simulink model "DTFC_SVM"  (R2019b)
settings: Solver=VariableStepAuto  StartTime=0.0  StopTime=15  RelTol=1e-3
undefined symbols (not defined in the file or in its folder): find_system, psisx, Rs, Ts, Ts_SVPWM, Vdc
libraries: powerlib x15, powerlib_meascontrol x3, simulink_extras x3, simulink x2
settings Model: Creator=ADHI  LastModifiedBy=ADHI
settings DataIOCC: ReturnWorkspaceOutputs=off
settings DebuggingCC: ArithmeticOperatorsInVariantConditions=warning
settings SFSimCC: SimUseLocalCustomCode=off  CustomCodeUndefinedFunction=UseInterfaceOnly
settings RTWCC: RTWUseLocalCustomCode=off

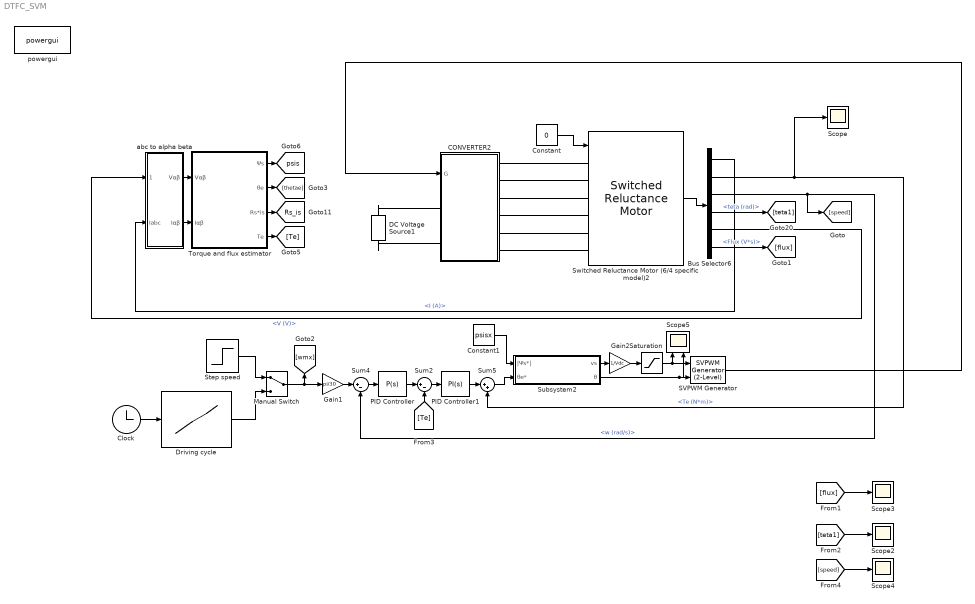
== system DTFC_SVM ==
  Bus Selector6 : BusSelector  OutputSignals=I (A),Te (N*m),w (rad/s),teta (rad),V (V),Flux (V*s)
  CONVERTER2 : Subsystem  LoadFcn=find_system(gcs,'FollowLinks', 'on', 'LookUnderMasks', 'all');
  Clock : Clock
  Constant : Constant  Value=0
  Constant1 : Constant  Value=psisx
  DC Voltage Source1 : powerlib/Electrical Sources/DC Voltage Source  Amplitude=250  Measurements=None
      settings: SourceProductName=Simscape Electrical
  Driving cycle : Lookup_n-D  NumberOfTableDimensions=1  BreakpointsForDimension1=[0 1 2 5 5.001 8 8.001 10 11 12]/2  Table=[0 0 480 480 1430 1430 0 0 480 480]  RndMeth=Simplest  InputSameDT=on
  Gain1 : Gain  Gain=pi/30
  Gain2 : Gain  Gain=1/Vdc
  Manual Switch : ManualSwitch
  PID Controller : simulink/Continuous/PID Controller  Controller=P  Form=Parallel  TimeDomain=Continuous-time  SampleTime=-1  IntegratorMethod=Forward Euler  FilterMethod=Forward Euler  ControllerParametersSource=internal  P=20  I=20  D=0  UseFilter=on  N=100  TunerSelectOption=Transfer Function Based (PID Tuner App)  InitialConditionSource=internal  InitialConditionForIntegrator=0  InitialConditionForFilter=0  DifferentiatorICPrevScaledInput=0  ExternalReset=none  TrackingMode=off  Kt=1  LimitOutput=on  UpperSaturationLimit=30  LowerSaturationLimit=-30  LinearizeAsGain=on  AntiWindupMode=clamping  Kb=1  POutMin=[]  POutMax=[]  IOutMin=[]  IOutMax=[]  DOutMin=[]  DOutMax=[]  NOutMin=[]  NOutMax=[]  SumOutMin=[]  SumOutMax=[]  SaturationOutMin=[]  SaturationOutMax=[]  PParamMin=[]  PParamMax=[]  IParamMin=[]  IParamMax=[]  DParamMin=[]  DParamMax=[]  NParamMin=[]  NParamMax=[]  KbParamMin=[]  KbParamMax=[]  KtParamMin=[]  KtParamMax=[]  KbOutMin=[]  KbOutMax=[]  KtOutMin=[]  KtOutMax=[]  IntegratorOutMin=[]  IntegratorOutMax=[]  FilterOutMin=[]  FilterOutMax=[]  SumI1OutMin=[]  SumI1OutMax=[]  SumI2OutMin=[]  SumI2OutMax=[]  SumI3OutMin=[]  SumI3OutMax=[]  SumI4OutMin=[]  SumI4OutMax=[]  SumDOutMin=[]  SumDOutMax=[]  DifferentiatorOutMin=[]  DifferentiatorOutMax=[]  FilterDiffOutCoefMin=[]  FilterDiffOutCoefMax=[]  ReciprocalOutMin=[]  ReciprocalOutMax=[]  SumDenOutMin=[]  SumDenOutMax=[]  SumNumOutMin=[]  SumNumOutMax=[]  DivideOutMin=[]  DivideOutMax=[]  IntegratorContinuousStateAttributes=''  IntegratorStateMustResolveToSignalObject=off  IntegratorRTWStateStorageClass=Auto  FilterContinuousStateAttributes=''  FilterStateMustResolveToSignalObject=off  FilterRTWStateStorageClass=Auto  ParallelPVariant=InternalParameters  IdealPVariant=Disabled  IVariant=Disabled  DVariant=Disabled  IntegratorVariant=Disabled  SatVariant=Enabled  AWVariant=Disabled  PCopyVariant=Disabled  TRVariant=Disabled  FdbkBlocksVariant=Forward  IdealPFdbkVariant=Disabled  SatFdbkVariant=Disabled  DerivativeFilterVariant=Disabled  NVariant=Disabled  NCopyVariant=Disabled_SignalSpec  FilterICVariant=Disabled  IntegratorICVariant=Disabled  ExternalResetVariant=Disabled  TRSumVariant=Passthrough  SumFdbkVariant=Disabled  SumVariant=Passthrough_P
  PID Controller1 : simulink/Continuous/PID Controller  Controller=PI  Form=Parallel  TimeDomain=Continuous-time  SampleTime=-1  IntegratorMethod=Forward Euler  FilterMethod=Forward Euler  ControllerParametersSource=internal  P=0.005  I=1  D=0.00005  UseFilter=on  N=100  TunerSelectOption=Transfer Function Based (PID Tuner App)  InitialConditionSource=internal  InitialConditionForIntegrator=0  InitialConditionForFilter=0  DifferentiatorICPrevScaledInput=0  ExternalReset=none  TrackingMode=off  Kt=1  LimitOutput=on  UpperSaturationLimit=pi/2  LowerSaturationLimit=-pi/2  LinearizeAsGain=on  AntiWindupMode=clamping  Kb=1  POutMin=[]  POutMax=[]  IOutMin=[]  IOutMax=[]  DOutMin=[]  DOutMax=[]  NOutMin=[]  NOutMax=[]  SumOutMin=[]  SumOutMax=[]  SaturationOutMin=[]  SaturationOutMax=[]  PParamMin=[]  PParamMax=[]  IParamMin=[]  IParamMax=[]  DParamMin=[]  DParamMax=[]  NParamMin=[]  NParamMax=[]  KbParamMin=[]  KbParamMax=[]  KtParamMin=[]  KtParamMax=[]  KbOutMin=[]  KbOutMax=[]  KtOutMin=[]  KtOutMax=[]  IntegratorOutMin=[]  IntegratorOutMax=[]  FilterOutMin=[]  FilterOutMax=[]  SumI1OutMin=[]  SumI1OutMax=[]  SumI2OutMin=[]  SumI2OutMax=[]  SumI3OutMin=[]  SumI3OutMax=[]  SumI4OutMin=[]  SumI4OutMax=[]  SumDOutMin=[]  SumDOutMax=[]  DifferentiatorOutMin=[]  DifferentiatorOutMax=[]  FilterDiffOutCoefMin=[]  FilterDiffOutCoefMax=[]  ReciprocalOutMin=[]  ReciprocalOutMax=[]  SumDenOutMin=[]  SumDenOutMax=[]  SumNumOutMin=[]  SumNumOutMax=[]  DivideOutMin=[]  DivideOutMax=[]  IntegratorContinuousStateAttributes=''  IntegratorStateMustResolveToSignalObject=off  IntegratorRTWStateStorageClass=Auto  FilterContinuousStateAttributes=''  FilterStateMustResolveToSignalObject=off  FilterRTWStateStorageClass=Auto  ParallelPVariant=InternalParameters  IdealPVariant=Disabled  IVariant=InternalParameters  DVariant=Disabled  IntegratorVariant=Continuous  SatVariant=Enabled  AWVariant=ContClampingParallel  PCopyVariant=Disabled  TRVariant=Disabled  FdbkBlocksVariant=Forward  IdealPFdbkVariant=Disabled  SatFdbkVariant=Disabled  DerivativeFilterVariant=Disabled  NVariant=Disabled  NCopyVariant=Disabled_SignalSpec  FilterICVariant=Disabled  IntegratorICVariant=InternalICs  ExternalResetVariant=Disabled  TRSumVariant=Passthrough  SumFdbkVariant=Disabled  SumVariant=Sum_PI
  SVPWM Generator : powerlib_meascontrol/Pulse & Signal Generators/SVPWM Generator (2-Level)  InputType=Magnitude-Angle (rad)  SwitchingPattern=Pattern #1  Fc=1/Ts_SVPWM  ParUref=[0.8 -30 50]  Ts=Ts
      settings: SourceProductName=Simscape Electrical  SourceProductBaseCode=PS
  Saturation : Saturate  UpperLimit=1  LowerLimit=0
  Scope{,2..4} (4 alike) : Scope
  Scope5 : Scope  NumInputPorts=2
  Step speed : Step  Time=0.15  After=1200  SampleTime=0
  Subsystem2 : Subsystem
  Sum2 : Sum  Inputs=|+-
  Sum4 : Sum  Inputs=|+-  SaturateOnIntegerOverflow=on  InputSameDT=on  OutDataTypeStr=Inherit: Same as first input
  Sum5 : Sum  Inputs=|++
  Switched Reluctance Motor (6/4 specific model)2 : powerlib/Machines/Switched Reluctance Motor  MachineType=6/4  StatorResistance=0.05  Inertia=0.05  Friction=0.02  InitialSpeed=[0,0]  TsPowergui=0  TsBlock=Ts  MachineModel=Specific model  Lq=0.67e-3  Ld=23.6e-3  Lsat=0.15e-3  MaximumCurrent=450  MaximumFluxLinkage=0.486  Source=Dialog  MagnetisationCharacteristic=FTBL  RotorAngleVector=RotorAngles  StatorCurrentVector=StatorCurrents  PlotCurves=off
      settings: SourceProductName=Simscape Electrical  SourceProductBaseCode=PS
  Torque and flux estimator : Subsystem
  abc to alpha beta : Subsystem
  powergui : powerlib/powergui  Priority=1  SimulationMode=Discrete  SampleTime=Ts  frequency=60  Iterations=50  frequencyindice=0  Pbase=100e6  ErrMax=1e-4  UnitsV=kV  UnitsW=MW  buscounter=0  FunctionMessages=off  echomessages=off  EnableUseOfTLC=off  CurrentSourceSwitches=off  DisableSnubberDevices=off  DisableRonSwitches=off  DisableVfSwitches=off  DisplayEquations=off  AutomaticDiscreteSolvers=off  SolverType=Tustin/Backward Euler (TBE)  Interpol=off  ExternalGateDelay=off  methode=off  Ts=100  x0status=blocks  SPID=off  SwTol=0  HookPort=off  NonlinearTolerance=1e-4  nMaxIteration=100  ContinueOnMaxIteration=off  RestoreLinks=warning  ResistiveCurrentMeasurement=off  Frange=[0:2:500]  Ylog=off  Xlog=on  ShowGrid=off  save=off  variable=ZData  structure=0  ZoomFFT=off  StartTime=0.0  cycles=1  DisplayStyle=1  fundamental=60  FreqAxis=off  MaxFrequency=1000  frequencyindicesteady=1  RmsSteady=1  display=off
      settings: SourceProductName=Simscape Electrical
  tag scope: Rs_is=global, psis=global
  wires:
  SVPWM Generator/1 -> CONVERTER2/1(G)
  Switched Reluctance Motor (6/4 specific model)2/1 -> Bus Selector6/1
  Bus Selector6/1 -> abc to alpha beta/2(Iabc)  "<I (A)>"
  Bus Selector6/5 -> abc to alpha beta/1(Vabc)  "<V (V)>"
  Bus Selector6/4 -> [teta1]  "<teta (rad)>"
  Bus Selector6/3 -> [speed], Sum4/2  "<w (rad/s)>"
  Bus Selector6/2 -> Scope/1, Sum5/2  "<Te (N*m)>"
  Gain2/1 -> Saturation/1
  Sum5/1 -> Subsystem2/2(θe*)
  Sum4/1 -> PID Controller/1
  Torque and flux estimator/2(θe) -> [thetae]
  Driving cycle/1 -> Manual Switch/2
  abc to alpha beta/1(Vαβ) -> Torque and flux estimator/1(Vαβ)
  Torque and flux estimator/4(Te) -> [Te]
  Clock/1 -> Driving cycle/1
  Torque and flux estimator/1(Ψs) -> [psis]
  Torque and flux estimator/3(Rs*is) -> [Rs_is]
  Sum2/1 -> PID Controller1/1
  Constant1/1 -> Subsystem2/1(|Ψs*|)
  [Te] -> Sum2/2
  Subsystem2/1(vs) -> Gain2/1
  PID Controller1/1 -> Sum5/1
  Gain1/1 -> Sum4/1
  Manual Switch/1 -> [wmx], Gain1/1
  abc to alpha beta/2(Iαβ) -> Torque and flux estimator/2(Iαβ)
  Step speed/1 -> Manual Switch/1
  Saturation/1 -> SVPWM Generator/1, Scope5/1
  PID Controller/1 -> Sum2/1
  Subsystem2/2(θ) -> Scope5/2, SVPWM Generator/2
  Constant/1 -> Switched Reluctance Motor (6/4 specific model)2/1
  Bus Selector6/6 -> [flux]  "<Flux (V*s)>"
  [flux] -> Scope3/1
  [teta1] -> Scope2/1
  [speed] -> Scope4/1
  connections:
  CONVERTER2/RConn1 -- Switched Reluctance Motor (6/4 specific model)2/LConn1
  CONVERTER2/RConn2 -- Switched Reluctance Motor (6/4 specific model)2/LConn2
  CONVERTER2/RConn3 -- Switched Reluctance Motor (6/4 specific model)2/LConn3
  CONVERTER2/RConn4 -- Switched Reluctance Motor (6/4 specific model)2/LConn4
  CONVERTER2/RConn5 -- Switched Reluctance Motor (6/4 specific model)2/LConn5
  CONVERTER2/RConn6 -- Switched Reluctance Motor (6/4 specific model)2/LConn6
  DC Voltage Source1/RConn1 -- CONVERTER2/LConn1
  DC Voltage Source1/LConn1 -- CONVERTER2/LConn2

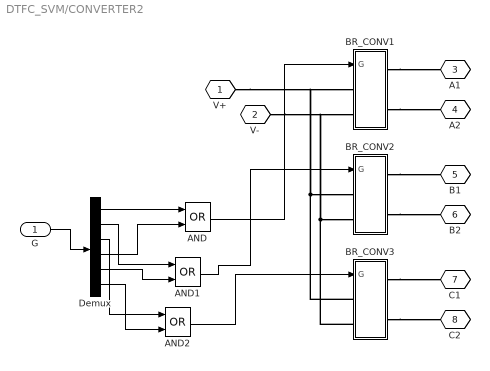
== system DTFC_SVM/CONVERTER2 ==
  G : Inport
  AND : Logic  Operator=OR  AllPortsSameDT=off  OutDataTypeStr=boolean
  AND1 : Logic  Operator=OR  AllPortsSameDT=off  OutDataTypeStr=boolean
  AND2 : Logic  Operator=OR  AllPortsSameDT=off  OutDataTypeStr=boolean
  BR_CONV1 : Subsystem
  BR_CONV2 : Subsystem
  BR_CONV3 : Subsystem
  Demux : Demux  Outputs=6
  V+ : PMIOPort  Tag=PMCPort  Side=Left
  V- : PMIOPort  Tag=PMCPort  Port=2  Side=Left
  A1 : PMIOPort  Tag=PMCPort  Port=3  Side=Right
  A2 : PMIOPort  Tag=PMCPort  Port=4  Side=Right
  B1 : PMIOPort  Tag=PMCPort  Port=5  Side=Right
  B2 : PMIOPort  Tag=PMCPort  Port=6  Side=Right
  C1 : PMIOPort  Tag=PMCPort  Port=7  Side=Right
  C2 : PMIOPort  Tag=PMCPort  Port=8  Side=Right
  wires:
  G/1 -> Demux/1
  AND/1 -> BR_CONV1/1(G)
  AND1/1 -> BR_CONV2/1(G)
  AND2/1 -> BR_CONV3/1(G)
  Demux/1 -> AND/1
  Demux/4 -> AND/2
  Demux/2 -> AND1/1
  Demux/3 -> AND2/1
  Demux/5 -> AND1/2
  Demux/6 -> AND2/2
  connections:
  BR_CONV3/RConn2 -- C2/RConn1
  BR_CONV3/RConn1 -- C1/RConn1
  BR_CONV2/RConn2 -- B2/RConn1
  BR_CONV2/RConn1 -- B1/RConn1
  BR_CONV1/RConn2 -- A2/RConn1
  BR_CONV1/RConn1 -- A1/RConn1
  BR_CONV3/LConn2 -- BR_CONV1/LConn2 -- V-/RConn1 -- BR_CONV2/LConn2
  BR_CONV3/LConn1 -- BR_CONV1/LConn1 -- V+/RConn1 -- BR_CONV2/LConn1

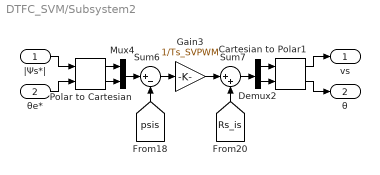
== system DTFC_SVM/Subsystem2 ==
  |Ψs*| : Inport
  θe* : Inport  Port=2
  Cartesian to Polar1 : simulink_extras/Transformations/Cartesian to Polar
      settings: SourceProductName=Simulink
  Demux2 : Demux  Outputs=2
  Gain3 : Gain  Gain=1/Ts_SVPWM
  Mux4 : Mux  Inputs=2
  Polar to Cartesian : simulink_extras/Transformations/Polar to Cartesian
      settings: SourceProductName=Simulink  SourceProductBaseCode=SL
  Sum6 : Sum  Inputs=|+-
  Sum7 : Sum  Inputs=|++
  vs : Outport  VectorParamsAs1DForOutWhenUnconnected=off
  θ : Outport  Port=2  VectorParamsAs1DForOutWhenUnconnected=off
  wires:
  Mux4/1 -> Sum6/1
  |Ψs*|/1 -> Polar to Cartesian/1
  Gain3/1 -> Sum7/1
  Polar to Cartesian/2 -> Mux4/2
  Demux2/1 -> Cartesian to Polar1/1
  Sum6/1 -> Gain3/1
  Demux2/2 -> Cartesian to Polar1/2
  [psis] -> Sum6/2
  Polar to Cartesian/1 -> Mux4/1
  Sum7/1 -> Demux2/1
  [Rs_is] -> Sum7/2
  θe*/1 -> Polar to Cartesian/2
  Cartesian to Polar1/1 -> vs/1
  Cartesian to Polar1/2 -> θ/1

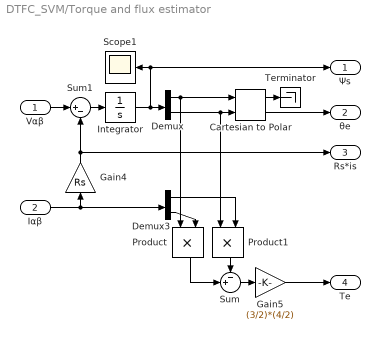
== system DTFC_SVM/Torque and flux estimator ==
  Vαβ : Inport
  Iαβ : Inport  Port=2
  Cartesian to Polar : simulink_extras/Transformations/Cartesian to Polar
      settings: SourceProductName=Simulink
  Demux : Demux  Outputs=2
  Demux3 : Demux  Outputs=2
  Gain4 : Gain  Gain=Rs
  Gain5 : Gain  Gain=(3/2)*(4/2)
  Integrator : Integrator
  Product : Product
  Product1 : Product
  Scope1 : Scope
  Sum : Sum  Inputs=-+|
  Sum1 : Sum  Inputs=|+-
  Terminator : Terminator
  Ψs : Outport  VectorParamsAs1DForOutWhenUnconnected=off
  θe : Outport  Port=2  VectorParamsAs1DForOutWhenUnconnected=off
  Rs*is : Outport  Port=3  VectorParamsAs1DForOutWhenUnconnected=off
  Te : Outport  Port=4  VectorParamsAs1DForOutWhenUnconnected=off
  wires:
  Vαβ/1 -> Sum1/1
  Integrator/1 -> Demux/1, Ψs/1, Scope1/1
  Sum1/1 -> Integrator/1
  Gain4/1 -> Rs*is/1, Sum1/2
  Demux3/1 -> Product1/2
  Demux3/2 -> Product/2
  Demux/2 -> Product1/1, Cartesian to Polar/2
  Product/1 -> Sum/2
  Cartesian to Polar/1 -> Terminator/1
  Demux/1 -> Cartesian to Polar/1, Product/1
  Sum/1 -> Gain5/1
  Product1/1 -> Sum/1
  Iαβ/1 -> Demux3/1, Gain4/1
  Gain5/1 -> Te/1
  Cartesian to Polar/2 -> θe/1

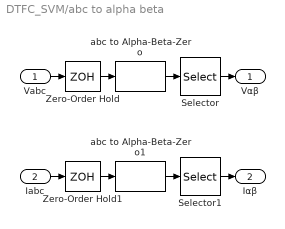
== system DTFC_SVM/abc to alpha beta ==
  Vabc : Inport
  Iabc : Inport  Port=2
  Selector : Selector  InputPortWidth=3  IndexOptions=Index vector (dialog)  Indices=[1 2]  OutputSizes=1
  Selector1 : Selector  InputPortWidth=3  IndexOptions=Index vector (dialog)  Indices=[1 2]  OutputSizes=1
  Zero-Order Hold : ZeroOrderHold  SampleTime=Ts
  Zero-Order Hold1 : ZeroOrderHold  SampleTime=Ts
  abc to Alpha-Beta-Zero : powerlib_meascontrol/Transformations/abc to Alpha-Beta-Zero
      settings: SourceProductName=Simscape Electrical
  abc to Alpha-Beta-Zero1 : powerlib_meascontrol/Transformations/abc to Alpha-Beta-Zero
      settings: SourceProductName=Simscape Electrical
  Vαβ : Outport  VectorParamsAs1DForOutWhenUnconnected=off
  Iαβ : Outport  Port=2  VectorParamsAs1DForOutWhenUnconnected=off
  wires:
  abc to Alpha-Beta-Zero/1 -> Selector/1
  Selector1/1 -> Iαβ/1
  Zero-Order Hold/1 -> abc to Alpha-Beta-Zero/1
  Vabc/1 -> Zero-Order Hold/1
  Selector/1 -> Vαβ/1
  Iabc/1 -> Zero-Order Hold1/1
  Zero-Order Hold1/1 -> abc to Alpha-Beta-Zero1/1
  abc to Alpha-Beta-Zero1/1 -> Selector1/1

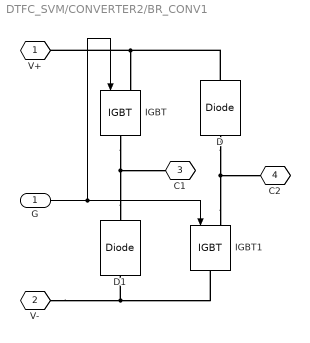
== system DTFC_SVM/CONVERTER2/BR_CONV1 ==
  G : Inport
  D : powerlib/Power Electronics/Diode  Ron=1e-3  Lon=0  Vf=0.8  IC=0  UseSnubber=off  Rs=1000  Cs=inf  Measurements=off
      settings: SourceProductName=Simscape Electrical
  D1 : powerlib/Power Electronics/Diode  Ron=1e-3  Lon=0  Vf=0.8  IC=0  UseSnubber=off  Rs=1000  Cs=inf  Measurements=off
      settings: SourceProductName=Simscape Electrical
  IGBT : powerlib/Power Electronics/IGBT  Ron=1e-3  Lon=0  Vf=1  Tf=0  Tt=0  IC=0  Rs=200  Cs=0.1e-6  Measurements=off
      settings: SourceProductName=Simscape Electrical
  IGBT1 : powerlib/Power Electronics/IGBT  Ron=1e-3  Lon=0  Vf=1  Tf=0  Tt=0  IC=0  Rs=200  Cs=0.1e-6  Measurements=off
      settings: SourceProductName=Simscape Electrical
  V+ : PMIOPort  Tag=PMCPort  Side=Left
  V- : PMIOPort  Tag=PMCPort  Port=2  Side=Left
  C1 : PMIOPort  Tag=PMCPort  Port=3  Side=Right
  C2 : PMIOPort  Tag=PMCPort  Port=4  Side=Right
  wires:
  G/1 -> IGBT/1, IGBT1/1
  connections:
  D1/LConn1 -- V-/RConn1 -- IGBT1/RConn1
  IGBT1/LConn1 -- D/LConn1 -- C2/RConn1
  D1/RConn1 -- IGBT/RConn1 -- C1/RConn1
  D/RConn1 -- V+/RConn1 -- IGBT/LConn1

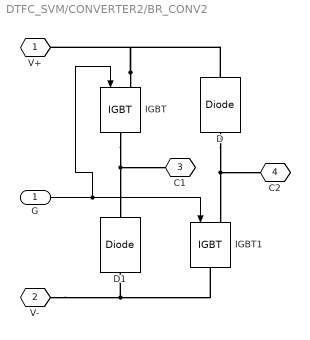
== system DTFC_SVM/CONVERTER2/BR_CONV2 ==
  G : Inport
  D : powerlib/Power Electronics/Diode  Ron=1e-3  Lon=0  Vf=0.8  IC=0  UseSnubber=off  Rs=1000  Cs=inf  Measurements=off
      settings: SourceProductName=Simscape Electrical
  D1 : powerlib/Power Electronics/Diode  Ron=1e-3  Lon=0  Vf=0.8  IC=0  UseSnubber=off  Rs=1000  Cs=inf  Measurements=off
      settings: SourceProductName=Simscape Electrical
  IGBT : powerlib/Power Electronics/IGBT  Ron=1e-3  Lon=0  Vf=1  Tf=0  Tt=0  IC=0  Rs=200  Cs=0.1e-6  Measurements=off
      settings: SourceProductName=Simscape Electrical
  IGBT1 : powerlib/Power Electronics/IGBT  Ron=1e-3  Lon=0  Vf=1  Tf=0  Tt=0  IC=0  Rs=200  Cs=0.1e-6  Measurements=off
      settings: SourceProductName=Simscape Electrical
  V+ : PMIOPort  Tag=PMCPort  Side=Left
  V- : PMIOPort  Tag=PMCPort  Port=2  Side=Left
  C1 : PMIOPort  Tag=PMCPort  Port=3  Side=Right
  C2 : PMIOPort  Tag=PMCPort  Port=4  Side=Right
  wires:
  G/1 -> IGBT/1, IGBT1/1
  connections:
  IGBT/LConn1 -- V+/RConn1 -- D/RConn1
  IGBT/RConn1 -- D1/RConn1 -- C1/RConn1
  D/LConn1 -- IGBT1/LConn1 -- C2/RConn1
  V-/RConn1 -- D1/LConn1 -- IGBT1/RConn1

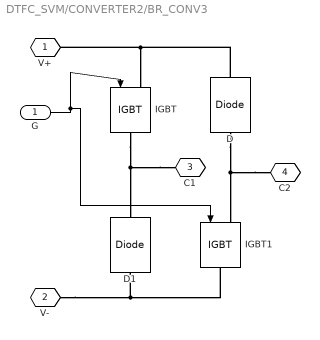
== system DTFC_SVM/CONVERTER2/BR_CONV3 ==
  G : Inport
  D : powerlib/Power Electronics/Diode  Ron=1e-3  Lon=0  Vf=0.8  IC=0  UseSnubber=off  Rs=1000  Cs=inf  Measurements=off
      settings: SourceProductName=Simscape Electrical
  D1 : powerlib/Power Electronics/Diode  Ron=1e-3  Lon=0  Vf=0.8  IC=0  UseSnubber=off  Rs=1000  Cs=inf  Measurements=off
      settings: SourceProductName=Simscape Electrical
  IGBT : powerlib/Power Electronics/IGBT  Ron=1e-3  Lon=0  Vf=1  Tf=0  Tt=0  IC=0  Rs=200  Cs=0.1e-6  Measurements=off
      settings: SourceProductName=Simscape Electrical
  IGBT1 : powerlib/Power Electronics/IGBT  Ron=1e-3  Lon=0  Vf=1  Tf=0  Tt=0  IC=0  Rs=200  Cs=0.1e-6  Measurements=off
      settings: SourceProductName=Simscape Electrical
  V+ : PMIOPort  Tag=PMCPort  Side=Left
  V- : PMIOPort  Tag=PMCPort  Port=2  Side=Left
  C1 : PMIOPort  Tag=PMCPort  Port=3  Side=Right
  C2 : PMIOPort  Tag=PMCPort  Port=4  Side=Right
  wires:
  G/1 -> IGBT1/1, IGBT/1
  connections:
  IGBT1/RConn1 -- D1/LConn1 -- V-/RConn1
  C2/RConn1 -- IGBT1/LConn1 -- D/LConn1
  C1/RConn1 -- D1/RConn1 -- IGBT/RConn1
  D/RConn1 -- V+/RConn1 -- IGBT/LConn1
